simulink model "Part3_1"  (R2021a)
settings: Solver=VariableStepAuto  StartTime=0.0  StopTime=100  RelTol=1e-3
settings Model: Creator=theod  LastModifiedBy=theod

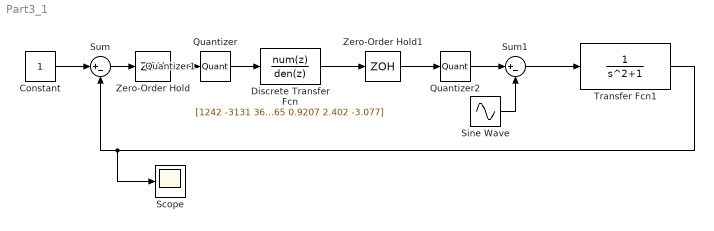
== system Part3_1 ==
  Constant : Constant
  Discrete Transfer Fcn : DiscreteTransferFcn  Numerator=[1242 -3131 3696 -2322 615.9]  Denominator=[1 1.919 -3.165 0.9207 2.402 -3.077]
  Quantizer : Quantizer
  Quantizer1 : Quantizer  QuantizationInterval=0.001
  Quantizer2 : Quantizer  QuantizationInterval=0.001
  Scope : Scope
  Sine Wave : Sin  Frequency=10  SampleTime=0
  Sum : Sum  Inputs=|+-
  Sum1 : Sum  Inputs=|+-
  Transfer Fcn1 : TransferFcn  Denominator=[1 0 1]
  Zero-Order Hold : ZeroOrderHold  SampleTime=0.1
  Zero-Order Hold1 : ZeroOrderHold  SampleTime=-1
  wires:
  Zero-Order Hold/1 -> Quantizer/1
  Discrete Transfer Fcn/1 -> Zero-Order Hold1/1
  Zero-Order Hold1/1 -> Quantizer2/1
  Sum/1 -> Zero-Order Hold/1
  Quantizer2/1 -> Sum1/1
  Sine Wave/1 -> Sum1/2
  Sum1/1 -> Transfer Fcn1/1
  Transfer Fcn1/1 -> Scope/1, Sum/2
  Constant/1 -> Sum/1
  Quantizer/1 -> Discrete Transfer Fcn/1
